simulink model "test_31_finalvrlload"  (R2013a)
settings: Solver=ode45  StartTime=0.0  StopTime=0.04  RelTol=1e-3
libraries: powerlib x35
settings Model: Creator=ies201042  LastModifiedBy=Administrator

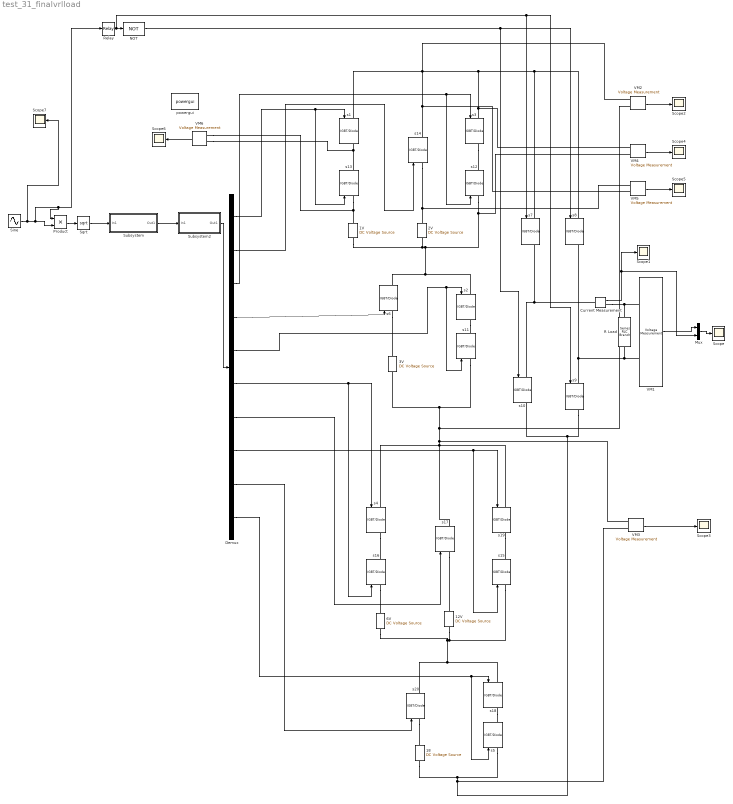
== system test_31_finalvrlload ==
  12V : powerlib/Electrical Sources/DC Voltage Source  Amplitude=8  Measurements=None
  18 : powerlib/Electrical Sources/DC Voltage Source  Amplitude=8  Measurements=None
  1V : powerlib/Electrical Sources/DC Voltage Source  Amplitude=1  Measurements=None
  2V : powerlib/Electrical Sources/DC Voltage Source  Amplitude=2  Measurements=None
  3V : powerlib/Electrical Sources/DC Voltage Source  Amplitude=2  Measurements=None
  6V : powerlib/Electrical Sources/DC Voltage Source  Amplitude=4  Measurements=None
  Current Measurement : powerlib/Measurements/Current Measurement  PhasorSimulation=off  OutputType=Complex  PSBequivalent=0
  Demux : Demux  Outputs=10
  Mux : Mux  Inputs=2
  NOT : Logic  Operator=NOT  AllPortsSameDT=off  OutDataTypeStr=boolean
  Product : Product
  R Load : powerlib/Elements/Series RLC Branch  LConnTagsString=__new0  RConnTagsString=__new0  BranchType=RL  Resistance=10  Inductance=20e-3  SetiL0=off  InitialCurrent=0  Capacitance=1e-6  Setx0=off  InitialVoltage=0  Measurements=None
  Relay : Relay  OnSwitchValue=0  OffSwitchValue=0
  Scope{,1..7} (8 alike) : Scope
      Scope settings: YMin=-40  YMax=40  SaveName=four_three_one
      Scope1 settings: YMin=-40  YMax=40  SaveName=four_three_one1
      Scope2 settings: YMin=-40  YMax=40  SaveName=four_three_one3
      Scope3 settings: YMin=-40  YMax=40  SaveName=four_three_one4
      Scope4 settings: YMin=-40  YMax=40  SaveName=four_three_one5
      Scope5 settings: YMin=-40  YMax=40  SaveName=four_three_one6
      Scope6 settings: YMin=-40  YMax=40  SaveName=four_three_one7
      Scope7 settings: YMin=-40  YMax=40  SaveName=four_three_one8  Decimation=50
  Sine : Sin  Amplitude=16  Frequency=2*pi*50  SampleTime=0
  Sqrt : Sqrt  SaturateOnIntegerOverflow=on
  Subsystem : Subsystem
  Subsystem2 : Subsystem
  VM{1..6} (6 alike) : powerlib/Measurements/Voltage Measurement  PhasorSimulation=off  OutputType=Complex  PSBequivalent=0
  powergui : powerlib/powergui  Priority=1  SimulationMode=Discrete  SolverType=Tustin  SampleTime=1e-6  frequency=60  SPID=off  DisableSnubberDevices=off  DisableRonSwitches=off  DisableVfSwitches=off  SwTol=0  Interpol=off  DisplayEquations=off  frequencyindice=0  Pbase=100e6  ErrMax=1e-4  Iterations=50  UnitsV=kV  UnitsW=MW  FunctionMessages=off  echomessages=off  HookPort=off  EnableUseOfTLC=off  x0status=blocks  RestoreLinks=warning  ResistiveCurrentMeasurement=off  Frange=[0:2:500]  Ylog=off  Xlog=on  ShowGrid=off  save=off  variable=ZData  structure=four_three_one1  ZoomFFT=off  StartTime=0.0  cycles=2  DisplayStyle=1  fundamental=50  FreqAxis=off  MaxFrequency=1000  frequencyindicesteady=1  RmsSteady=1  display=off  Ts=0  methode=off
  s{1..20} (20 alike) : powerlib/Power Electronics/IGBT//Diode  Ron=1e-3  Rs=1e5  Cs=inf  Measurements=on
  wires:
  VM1/1 -> Mux/1
  Sine/1 -> Scope7/1, Product/2, Relay/1, Product/1
  Subsystem/1(Out1) -> Subsystem2/1(In1)
  Product/1 -> Sqrt/1
  Sqrt/1 -> Subsystem/1(In1)
  Subsystem2/1(Out1) -> Demux/1
  NOT/1 -> s10/1, s8/1
  Relay/1 -> s9/1, s7/1, NOT/1
  Mux/1 -> Scope/1
  Current Measurement/1 -> Mux/2, Scope1/1
  Demux/1 -> s1/1, s13/1
  Demux/2 -> s14/1
  Demux/3 -> s12/1, s3/1
  Demux/6 -> s16/1, s4/1
  Demux/7 -> s17/1
  Demux/8 -> s15/1, s19/1
  Demux/9 -> s20/1
  Demux/10 -> s5/1, s18/1
  Demux/4 -> s6/1
  Demux/5 -> s11/1, s2/1
  VM2/1 -> Scope2/1
  VM3/1 -> Scope3/1
  VM4/1 -> Scope4/1
  VM5/1 -> Scope5/1
  VM6/1 -> Scope6/1
  connections:
  VM1/LConn1 -- Current Measurement/RConn1 -- R Load/LConn1
  s9/LConn1 -- s8/RConn1 -- VM1/LConn2 -- R Load/RConn1
  Current Measurement/LConn1 -- s10/LConn1 -- s7/RConn1
  3V/LConn1 -- VM3/LConn1 -- s4/LConn1 -- s19/LConn1 -- s17/RConn1 -- VM2/LConn2 -- s11/LConn1
  s6/LConn1 -- 3V/RConn1
  1V/LConn1 -- VM4/LConn2 -- s12/LConn1 -- s6/RConn1 -- s2/LConn1 -- 2V/LConn1
  s13/LConn1 -- VM6/LConn1 -- 1V/RConn1
  s14/LConn1 -- VM5/LConn1 -- 2V/RConn1
  s7/LConn1 -- s8/LConn1 -- VM4/LConn1 -- s3/LConn1 -- s1/LConn1 -- VM2/LConn1 -- s14/RConn1 -- VM5/LConn2
  s2/RConn1 -- s11/RConn1
  s1/RConn1 -- VM6/LConn2 -- s13/RConn1
  s3/RConn1 -- s12/RConn1
  s18/LConn1 -- s15/LConn1 -- 12V/LConn1 -- 6V/LConn1 -- s20/RConn1
  s4/RConn1 -- s16/RConn1
  s19/RConn1 -- s15/RConn1
  s17/LConn1 -- 12V/RConn1
  s16/LConn1 -- 6V/RConn1
  s20/LConn1 -- 18/RConn1
  s18/RConn1 -- s5/RConn1
  s9/RConn1 -- VM3/LConn2 -- 18/LConn1 -- s5/LConn1 -- s10/RConn1

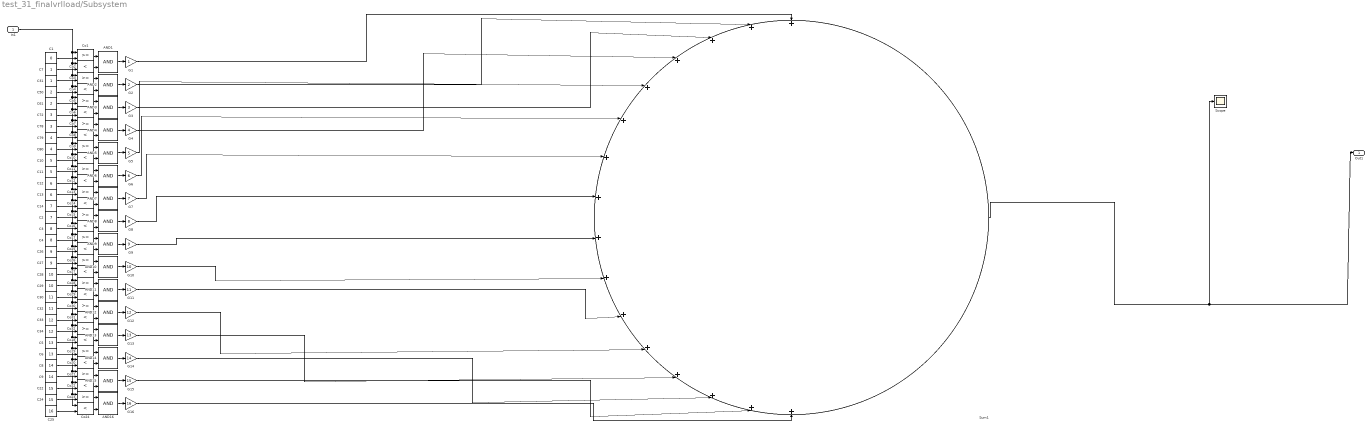
== system test_31_finalvrlload/Subsystem ==
  In1 : Inport
  AND{1..16} (16 alike) : Logic  AllPortsSameDT=off  OutDataTypeStr=boolean
  C1 : Constant  Value=0
  C10 : Constant  Value=5
  C11 : Constant  Value=5
  C12 : Constant  Value=6
  C13 : Constant  Value=6
  C14 : Constant  Value=7
  C2 : Constant  Value=7
  C22 : Constant  Value=15
  C24 : Constant  Value=15
  C25 : Constant  Value=16
  C26 : Constant  Value=9
  C27 : Constant  Value=9
  C28 : Constant  Value=10
  C29 : Constant  Value=10
  C3 : Constant  Value=8
  C30 : Constant  Value=11
  C31 : Constant
  C32 : Constant  Value=11
  C33 : Constant  Value=12
  C34 : Constant  Value=12
  C4 : Constant  Value=8
  C5 : Constant  Value=13
  C50 : Constant  Value=2
  C6 : Constant  Value=13
  C61 : Constant  Value=2
  C7 : Constant
  C72 : Constant  Value=3
  C78 : Constant  Value=3
  C79 : Constant  Value=4
  C8 : Constant  Value=14
  C80 : Constant  Value=4
  C9 : Constant  Value=14
  Co{1,3,5,7,9,11,13,15,17,19,21,23,26,28,30,32} (16 alike) : RelationalOperator  OutDataTypeStr=boolean
  Co{2,4,6,8,10,12,14,16,18,20,22,24..25,27,29,31} (16 alike) : RelationalOperator  Operator=<  OutDataTypeStr=boolean
  G1 : Gain
  G10 : Gain  Gain=10
  G11 : Gain  Gain=11
  G12 : Gain  Gain=12
  G13 : Gain  Gain=13
  G14 : Gain  Gain=14
  G15 : Gain  Gain=15
  G16 : Gain  Gain=16
  G2 : Gain  Gain=2
  G3 : Gain  Gain=3
  G4 : Gain  Gain=4
  G5 : Gain  Gain=5
  G6 : Gain  Gain=6
  G7 : Gain  Gain=7
  G8 : Gain  Gain=8
  G9 : Gain  Gain=9
  Scope : Scope
      settings: YMin=-40  YMax=40  SaveName=four_three_one2
  Sum1 : Sum  Inputs=++++++++++++++++
  Out1 : Outport
  wires:
  Co12/1 -> AND6/2
  AND8/1 -> G8/1
  Co2/1 -> AND1/2
  Co32/1 -> AND13/1
  Co1/1 -> AND1/1
  Co13/1 -> AND7/1
  C22/1 -> Co22/2
  Co18/1 -> AND13/2
  Co5/1 -> AND3/1
  Co31/1 -> AND12/2
  C14/1 -> Co14/2
  C72/1 -> Co6/2
  C26/1 -> Co25/2
  AND5/1 -> G5/1
  Co19/1 -> AND14/1
  C6/1 -> Co19/2
  AND16/1 -> G16/1
  C25/1 -> Co24/2
  C2/1 -> Co15/2
  AND1/1 -> G1/1
  Co11/1 -> AND6/1
  Co23/1 -> AND16/1
  AND13/1 -> G13/1
  AND11/1 -> G11/1
  C10/1 -> Co10/2
  C28/1 -> Co27/2
  Co30/1 -> AND12/1
  Co22/1 -> AND15/2
  C29/1 -> Co28/2
  C50/1 -> Co4/2
  C3/1 -> Co16/2
  C4/1 -> Co17/2
  AND2/1 -> G2/1
  C31/1 -> Co3/2
  Co29/1 -> AND11/2
  C13/1 -> Co13/2
  C30/1 -> Co29/2
  Co20/1 -> AND14/2
  C78/1 -> Co7/2
  C27/1 -> Co26/2
  AND10/1 -> G10/1
  C1/1 -> Co1/2
  C34/1 -> Co32/2
  Co17/1 -> AND9/1
  Co15/1 -> AND8/1
  C7/1 -> Co2/2
  C24/1 -> Co23/2
  C80/1 -> Co9/2
  Co6/1 -> AND3/2
  Co4/1 -> AND2/2
  Co3/1 -> AND2/1
  AND14/1 -> G14/1
  Co24/1 -> AND16/2
  AND12/1 -> G12/1
  Co9/1 -> AND5/1
  AND9/1 -> G9/1
  C11/1 -> Co11/2
  C9/1 -> Co21/2
  AND15/1 -> G15/1
  Co25/1 -> AND9/2
  C5/1 -> Co18/2
  AND7/1 -> G7/1
  Co21/1 -> AND15/1
  C12/1 -> Co12/2
  Co7/1 -> AND4/1
  Co8/1 -> AND4/2
  Co10/1 -> AND5/2
  AND6/1 -> G6/1
  AND4/1 -> G4/1
  Co27/1 -> AND10/2
  C8/1 -> Co20/2
  C32/1 -> Co30/2
  Co26/1 -> AND10/1
  C33/1 -> Co31/2
  Co16/1 -> AND8/2
  Co14/1 -> AND7/2
  AND3/1 -> G3/1
  C61/1 -> Co5/2
  Co28/1 -> AND11/1
  C79/1 -> Co8/2
  G16/1 -> Sum1/16
  G15/1 -> Sum1/15
  G14/1 -> Sum1/14
  G13/1 -> Sum1/13
  G12/1 -> Sum1/12
  G11/1 -> Sum1/11
  G10/1 -> Sum1/10
  G9/1 -> Sum1/9
  G8/1 -> Sum1/8
  G7/1 -> Sum1/7
  G6/1 -> Sum1/6
  G5/1 -> Sum1/5
  G4/1 -> Sum1/4
  G3/1 -> Sum1/3
  G2/1 -> Sum1/2
  G1/1 -> Sum1/1
  Sum1/1 -> Out1/1, Scope/1
  In1/1 -> Co3/1, Co4/1, Co5/1, Co6/1, Co7/1, Co8/1, Co9/1, Co10/1, Co11/1, Co12/1, Co13/1, Co14/1, Co15/1, Co16/1, Co17/1, Co25/1, Co26/1, Co27/1, Co28/1, Co29/1, Co30/1, Co31/1, Co32/1, Co18/1, Co19/1, Co20/1, Co21/1, Co22/1, Co23/1, Co24/1, Co2/1, Co1/1

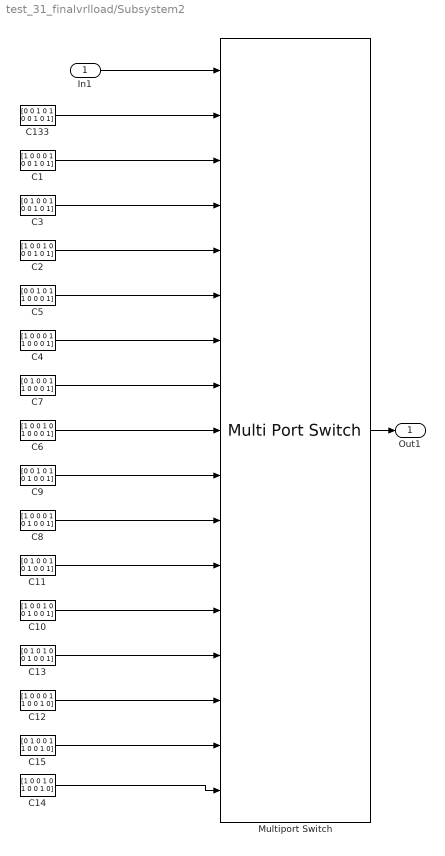
== system test_31_finalvrlload/Subsystem2 ==
  In1 : Inport
  C1 : Constant  Value=[1 0 0 0 1 0 0 1 0 1]
  C10 : Constant  Value=[1 0 0 1 0 0 1 0 0 1]
  C11 : Constant  Value=[0 1 0 0 1 0 1 0 0 1]
  C12 : Constant  Value=[1 0 0 0 1 1 0 0 1 0]
  C13 : Constant  Value=[0 1 0 1 0 0 1 0 0 1]
  C133 : Constant  Value=[0 0 1 0 1 0 0 1 0 1]
  C14 : Constant  Value=[1 0 0 1 0 1 0 0 1 0]
  C15 : Constant  Value=[0 1 0 0 1 1 0 0 1 0]
  C2 : Constant  Value=[1 0 0 1 0 0 0 1 0 1]
  C3 : Constant  Value=[0 1 0 0 1 0 0 1 0 1]
  C4 : Constant  Value=[1 0 0 0 1 1 0 0 0 1]
  C5 : Constant  Value=[0 0 1 0 1 1 0 0 0 1]
  C6 : Constant  Value=[1 0 0 1 0 1 0 0 0 1]
  C7 : Constant  Value=[0 1 0 0 1 1 0 0 0 1]
  C8 : Constant  Value=[1 0 0 0 1 0 1 0 0 1]
  C9 : Constant  Value=[0 0 1 0 1 0 1 0 0 1]
  Multiport Switch : MultiPortSwitch  Inputs=16  DiagnosticForDefault=None
  Out1 : Outport
  wires:
  In1/1 -> Multiport Switch/1
  Multiport Switch/1 -> Out1/1
  C133/1 -> Multiport Switch/2
  C2/1 -> Multiport Switch/5
  C3/1 -> Multiport Switch/4
  C1/1 -> Multiport Switch/3
  C5/1 -> Multiport Switch/6
  C10/1 -> Multiport Switch/13
  C8/1 -> Multiport Switch/11
  C13/1 -> Multiport Switch/14
  C15/1 -> Multiport Switch/16
  C7/1 -> Multiport Switch/8
  C11/1 -> Multiport Switch/12
  C6/1 -> Multiport Switch/9
  C4/1 -> Multiport Switch/7
  C12/1 -> Multiport Switch/15
  C9/1 -> Multiport Switch/10
  C14/1 -> Multiport Switch/17
